simulink model "llsy"  (R2018a)
settings: Solver=ode3  StartTime=0.0  StopTime=30  FixedStep=0.005  RelTol=1e-3  EnableMultiTasking=on
settings Model: Creator=Administrator  LastModifiedBy=xinxin
settings DataIOCC: LimitDataPoints=on  SaveFormat=Array
settings OptimizationCC: ExpressionDepthLimit=2147483647  LifeSpan=inf
settings DebuggingCC: UnderspecifiedInitializationDetection=Classic  MergeDetectMultiDrivingBlocksExec=none  SolverPrmCheckMsg=warning  FcnCallInpInsideContextMsg=warning  StateNameClashWarn=warning  SFUnexpectedBacktrackingDiag=warning  SFNoUnconditionalDefaultTransitionDiag=warning  SFExecutionAtInitializationDiag=none
settings HardwareCC: ProdBitPerPointer=32  ProdBitPerSizeT=32  ProdBitPerPtrDiffT=32  ProdLargestAtomicFloat=None  ProdIntDivRoundTo=Undefined  ProdEndianess=Unspecified  ProdWordSize=32  ProdHWDeviceType=32-bit Generic
settings ModelReferenceCC: PropagateSignalLabelsOutOfModel=off
settings CodeAppCC: StateflowObjectComments=on
settings GRTTargetCC: TargetLangStandard=C89/C90 (ANSI)  GeneratePreprocessorConditionals=Disable all
settings ConfigComp: CovMetricSettings=dw  CovHtmlReporting=on  CovSaveCumulativeToWorkspaceVar=on  CovSaveSingleToWorkspaceVar=on  CovExternalEMLEnable=off  CovSFcnEnable=off

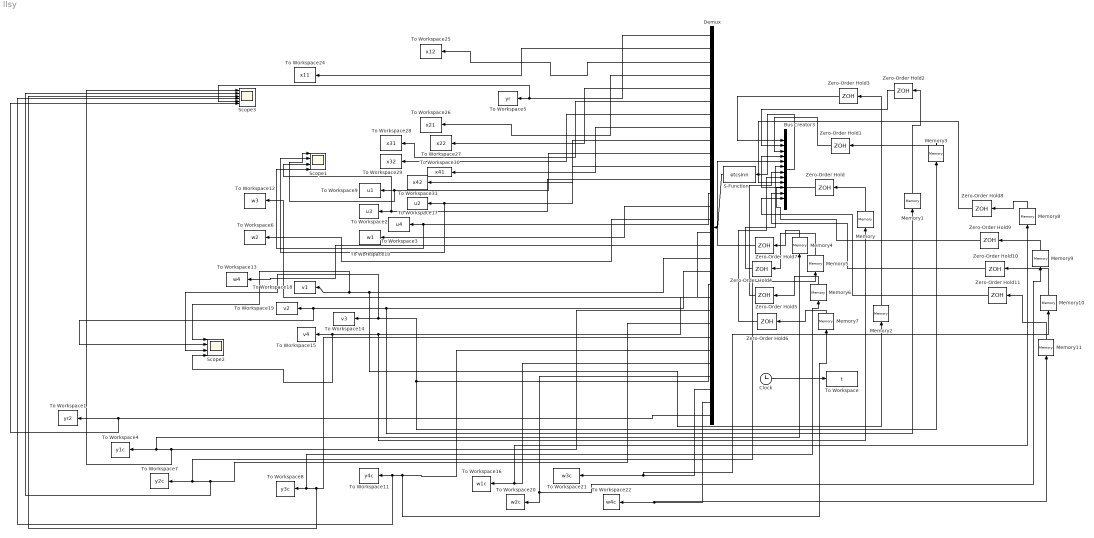
== system llsy ==
  Bus Creator3 : BusCreator  Inputs=12
  Clock : Clock
      settings: Decimation=20
  Demux : Demux  Outputs=30
  Memory{,4..11} (9 alike) : Memory  InheritSampleTime=on  LinearizeMemory=on  LinearizeAsDelay=on
  Memory1 : Memory
  Memory2 : Memory
  Memory3 : Memory
  S-Function : S-Function  FunctionName=etcsinn  SFunctionDeploymentMode=off  EnableBusSupport=off
  Scope1 : Scope  NumInputPorts=4
  Scope2 : Scope  NumInputPorts=4
  Scope3 : Scope  NumInputPorts=6
  To Workspace : ToWorkspace  VariableName=t  SampleTime=-1
  To Workspace1 : ToWorkspace  VariableName=yr2  SampleTime=-1
  To Workspace10 : ToWorkspace  VariableName=w1  SampleTime=-1
  To Workspace11 : ToWorkspace  VariableName=y4c  SampleTime=-1
  To Workspace12 : ToWorkspace  VariableName=w3  SampleTime=-1
  To Workspace13 : ToWorkspace  VariableName=w4  SampleTime=-1
  To Workspace14 : ToWorkspace  VariableName=v3  SampleTime=-1
  To Workspace15 : ToWorkspace  VariableName=v4  SampleTime=-1
  To Workspace16 : ToWorkspace  VariableName=w1c  SampleTime=-1
  To Workspace17 : ToWorkspace  VariableName=u2  SampleTime=-1
  To Workspace18 : ToWorkspace  VariableName=v1  SampleTime=-1
  To Workspace19 : ToWorkspace  VariableName=v2  SampleTime=-1
  To Workspace2 : ToWorkspace  VariableName=u3  SampleTime=-1
  To Workspace20 : ToWorkspace  VariableName=w2c  SampleTime=-1
  To Workspace21 : ToWorkspace  VariableName=w3c  SampleTime=-1
  To Workspace22 : ToWorkspace  VariableName=w4c  SampleTime=-1
  To Workspace24 : ToWorkspace  VariableName=x11  SampleTime=-1
  To Workspace25 : ToWorkspace  VariableName=x12  SampleTime=-1
  To Workspace26 : ToWorkspace  VariableName=x21  SampleTime=-1
  To Workspace27 : ToWorkspace  VariableName=x22  SampleTime=-1
  To Workspace28 : ToWorkspace  VariableName=x31  SampleTime=-1
  To Workspace29 : ToWorkspace  VariableName=x32  SampleTime=-1
  To Workspace3 : ToWorkspace  VariableName=u4  SampleTime=-1
  To Workspace30 : ToWorkspace  VariableName=x41  SampleTime=-1
  To Workspace31 : ToWorkspace  VariableName=x42  SampleTime=-1
  To Workspace4 : ToWorkspace  VariableName=y1c  SampleTime=-1
  To Workspace5 : ToWorkspace  VariableName=yr  SampleTime=-1
  To Workspace6 : ToWorkspace  VariableName=w2  SampleTime=-1
  To Workspace7 : ToWorkspace  VariableName=y2c  SampleTime=-1
  To Workspace8 : ToWorkspace  VariableName=y3c  SampleTime=-1
  To Workspace9 : ToWorkspace  VariableName=u1  SampleTime=-1
  Zero-Order Hold{,1..11} (12 alike) : ZeroOrderHold  SampleTime=0.005
  wires:
  Clock/1 -> To Workspace/1
  S-Function/1 -> Demux/1
  Bus Creator3/1 -> S-Function/1
  Memory1/1 -> Zero-Order Hold2/1
  Memory2/1 -> Zero-Order Hold3/1
  Memory3/1 -> Zero-Order Hold1/1
  Memory/1 -> Zero-Order Hold/1
  Zero-Order Hold1/1 -> Bus Creator3/3
  Zero-Order Hold/1 -> Bus Creator3/4
  Zero-Order Hold3/1 -> Bus Creator3/1
  Demux/1 -> Scope3/5, To Workspace5/1
  Demux/3 -> To Workspace25/1
  Demux/5 -> To Workspace27/1
  Demux/6 -> To Workspace28/1
  Demux/7 -> To Workspace29/1
  Demux/8 -> To Workspace30/1
  Demux/9 -> To Workspace31/1
  Demux/10 -> Scope1/1, To Workspace9/1
  Demux/11 -> Scope1/2, To Workspace17/1
  Demux/12 -> Scope1/3, To Workspace2/1
  Demux/13 -> Scope1/4, To Workspace3/1
  Demux/18 -> Memory2/1, Scope2/1, To Workspace18/1
  Demux/19 -> Memory1/1, Scope2/2, To Workspace19/1
  Demux/20 -> Scope2/3, To Workspace14/1, Memory3/1
  Demux/21 -> Memory/1, Scope2/4, To Workspace15/1
  Zero-Order Hold2/1 -> Bus Creator3/2
  Demux/2 -> To Workspace24/1
  Demux/4 -> To Workspace26/1
  Demux/14 -> To Workspace10/1
  Demux/15 -> To Workspace6/1
  Demux/16 -> To Workspace12/1
  Demux/17 -> To Workspace13/1
  Demux/27 -> Memory9/1, To Workspace20/1
  Demux/22 -> Scope3/1, Memory4/1, To Workspace4/1
  Demux/23 -> Scope3/2, Memory5/1, To Workspace7/1
  Demux/24 -> Scope3/3, Memory6/1, To Workspace8/1
  Demux/25 -> Memory7/1, Scope3/4, To Workspace11/1
  Demux/26 -> Memory8/1, To Workspace16/1
  Demux/28 -> Memory10/1, To Workspace21/1
  Demux/29 -> Memory11/1, To Workspace22/1
  Demux/30 -> Scope3/6, To Workspace1/1
  Memory4/1 -> Zero-Order Hold7/1
  Zero-Order Hold7/1 -> Bus Creator3/5
  Zero-Order Hold4/1 -> Bus Creator3/6
  Memory5/1 -> Zero-Order Hold4/1
  Zero-Order Hold5/1 -> Bus Creator3/7
  Memory6/1 -> Zero-Order Hold5/1
  Zero-Order Hold6/1 -> Bus Creator3/8
  Memory7/1 -> Zero-Order Hold6/1
  Zero-Order Hold8/1 -> Bus Creator3/9
  Memory8/1 -> Zero-Order Hold8/1
  Zero-Order Hold9/1 -> Bus Creator3/10
  Memory9/1 -> Zero-Order Hold9/1
  Zero-Order Hold10/1 -> Bus Creator3/11
  Memory10/1 -> Zero-Order Hold10/1
  Zero-Order Hold11/1 -> Bus Creator3/12
  Memory11/1 -> Zero-Order Hold11/1
